simulink model "pend_swingup"  (Simulink 9.1)
settings: Solver=ode4  StartTime=0.0  StopTime=20  FixedStep=0.01  RelTol=1e-3  EnableMultiTasking=on
values from neighbouring files (symbols this model uses):
  K = lqr(As,Bs,Q,R)    [pend_state_estimator_init.m]
undefined symbols (not defined in the file or in its folder): a, b, c, c2, d, f, h, J2, Ksw
settings Model: Creator=HOME  LastModifiedBy=DELL
settings DataIOCC: LimitDataPoints=on  SignalLoggingSaveFormat=ModelDataLogs
settings OptimizationCC: ExpressionDepthLimit=2147483647
settings DebuggingCC: SaveWithParameterizedLinksMsg=none  SolverPrmCheckMsg=warning  MultiTaskCondExecSysMsg=none  FcnCallInpInsideContextMsg=warning  StateNameClashWarn=warning
settings GRTTargetCC: GeneratePreprocessorConditionals=Disable all

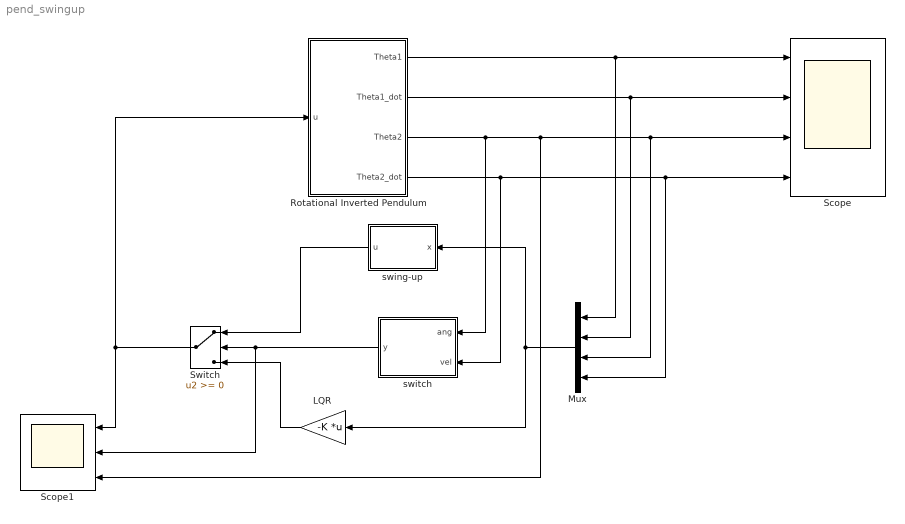
== system pend_swingup ==
  LQR : Gain  Gain=-K  Multiplication=Matrix(K*u)
  Mux : Mux
  Rotational Inverted Pendulum : Subsystem
  Scope : Scope  NumInputPorts=4
  Scope1 : Scope  NumInputPorts=3
  Switch : Switch
  swing-up : Subsystem
  switch : MATLAB Function  TreatAsAtomicUnit=on
  wires:
  Rotational Inverted Pendulum/1(Theta1) -> Scope/1, Mux/1
  Rotational Inverted Pendulum/2(Theta1_dot) -> Scope/2, Mux/2
  Rotational Inverted Pendulum/3(Theta2) -> Scope/3, Mux/3, Scope1/3, switch/1(ang)
  Rotational Inverted Pendulum/4(Theta2_dot) -> Scope/4, Mux/4, switch/2(vel)
  Mux/1 -> swing-up/1(x), LQR/1
  switch/1(y) -> Switch/2, Scope1/2
  LQR/1 -> Switch/3
  swing-up/1(u) -> Switch/1
  Switch/1 -> Rotational Inverted Pendulum/1(u), Scope1/1

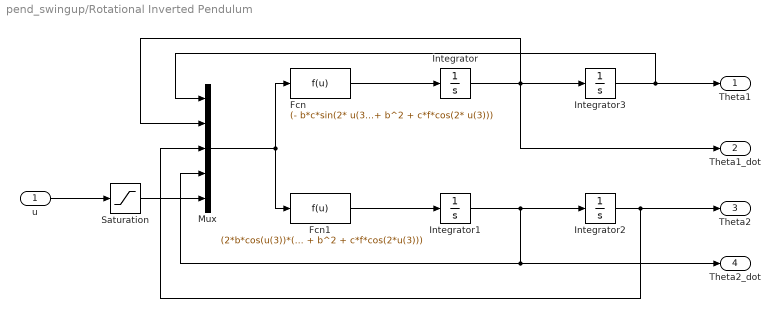
== system pend_swingup/Rotational Inverted Pendulum ==
  u : Inport
  Fcn : Fcn  Expr=(- b*c*sin(2* u(3))*cos(u(3))* u(2)^2 + 2*c*f*sin(2* u(3))* u(2)* u(4) + 2*d*f* u(2) + 2*b*f*sin(u(3))* u(4)^2 + 2*b*c2*cos(u(3))* u(4) - 2*e*f* u(5)- 2*b*h*cos(u(3))*sin(u(3)))/(b^2*cos(2* u(3)) - c*f - 2*a*f + b^2 + c*f*cos(2* u(3)))
  Fcn1 : Fcn  Expr=(2*b*cos(u(3))*(b*sin(u(3))*u(4)^2 + c*u(2)*sin(2*u(3))*u(4) + d*u(2) - e*u(5)))/(b^2*cos(2*u(3)) - c*f - 2*a*f + b^2 + c*f*cos(2*u(3))) - (((c*sin(2*u(3))*u(2)^2)/2 - c2*u(4) + h*sin(u(3)))*(2*a + c - c*cos(2*u(3))))/(b^2*cos(2*u(3)) - c*f - 2*a*f + b^2 + c*f*cos(2*u(3)))
  Integrator : Integrator
  Integrator1 : Integrator  InitialCondition=0.1
  Integrator2 : Integrator  InitialCondition=-pi
  Integrator3 : Integrator
  Mux : Mux  Inputs=5
  Saturation : Saturate  UpperLimit=25  LowerLimit=-25
  Theta1 : Outport
  Theta1_dot : Outport  Port=2
  Theta2 : Outport  Port=3
  Theta2_dot : Outport  Port=4
  wires:
  u/1 -> Saturation/1
  Saturation/1 -> Mux/5
  Mux/1 -> Fcn/1, Fcn1/1
  Fcn/1 -> Integrator/1
  Integrator/1 -> Integrator3/1, Theta1_dot/1, Mux/2
  Integrator3/1 -> Theta1/1, Mux/1
  Fcn1/1 -> Integrator1/1
  Integrator1/1 -> Integrator2/1, Theta2_dot/1, Mux/4
  Integrator2/1 -> Theta2/1, Mux/3

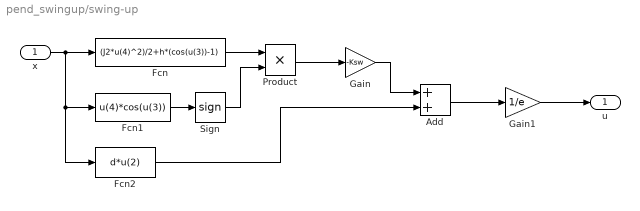
== system pend_swingup/swing-up ==
  x : Inport
  Add : Sum
  Fcn : Fcn  Expr=(J2*u(4)^2)/2+h*(cos(u(3))-1)
  Fcn1 : Fcn  Expr=u(4)*cos(u(3))
  Fcn2 : Fcn  Expr=d*u(2)
  Gain : Gain  Gain=-Ksw
  Gain1 : Gain  Gain=1/e
  Product : Product  RndMeth=Zero
  Sign : Signum
  u : Outport
  wires:
  x/1 -> Fcn/1, Fcn1/1, Fcn2/1
  Fcn1/1 -> Sign/1
  Fcn/1 -> Product/1
  Sign/1 -> Product/2
  Product/1 -> Gain/1
  Gain/1 -> Add/1
  Fcn2/1 -> Add/2
  Add/1 -> Gain1/1
  Gain1/1 -> u/1

== matlab function switch ==
  settings: fimath=|
      | fimath(...
      | 'RoundMode', 'floor',...
      | 'OverflowMode', 'wrap',...
      | 'ProductMode', 'KeepLSB', 'ProductWordLength', 32,...
      | 'SumMode', 'KeepLSB', 'SumWordLength', 32,...
      | 'CastBeforeSum', false)
  data: ang input double; y output double; vel input double
function y = switchC(ang, vel)

temp = mod(ang, 2*pi);
if(temp>pi)
temp=temp-2*pi;
end

if((abs(temp)<pi*20/180)&&(abs(vel)<2*pi))
y=-1;
else
y = 1;
end
